simulink model "csu_cmg_camera_geometry_hrn"  (R2014b)
settings: Solver=FixedStepDiscrete  StartTime=0  StopTime=1  FixedStep=1  RelTol=1e-3
values from neighbouring files (symbols this model uses):
  cam_extrinsic_init = zeros(3,4)    [csc_cam_camera_system_init.m]
  cam_image_plane_norm = [0 0 1]    [csc_cam_camera_system_init.m]
  topo_pos_in = [0 0 50+(central_body_radius + ini_alt_wrt_meanrad) ]    [csu_cmg_camera_geometry_test.m]
  topo_q_in = [0 0 sind(5/2) cosd(5/2)]    [csu_cmg_camera_geometry_test.m]
undefined symbols (not defined in the file or in its folder): cam_cam_lander_dcm, cam_intrinsic_matrix_c, cam_position_in_lander, cam_u_matrix, csu_cmg_camera_geometry, csu_cmg_camera_geometry_lib, ini_alt_wrt_1738rad, ini_tgt_landing_mcmf_pos
libraries: util_quat_lib x16, util_frame_rotation_lib x8, rotate_lib x2, util_common_lib x2
settings Model: Creator=escrane  LastModifiedBy=mstewart
settings DataIOCC: SignalLoggingSaveFormat=ModelDataLogs
settings OptimizationCC: ExpressionDepthLimit=2147483647
settings DebuggingCC: UnderspecifiedInitializationDetection=Classic  MergeDetectMultiDrivingBlocksExec=none  FcnCallInpInsideContextMsg=EnableAllAsWarning  StateNameClashWarn=warning

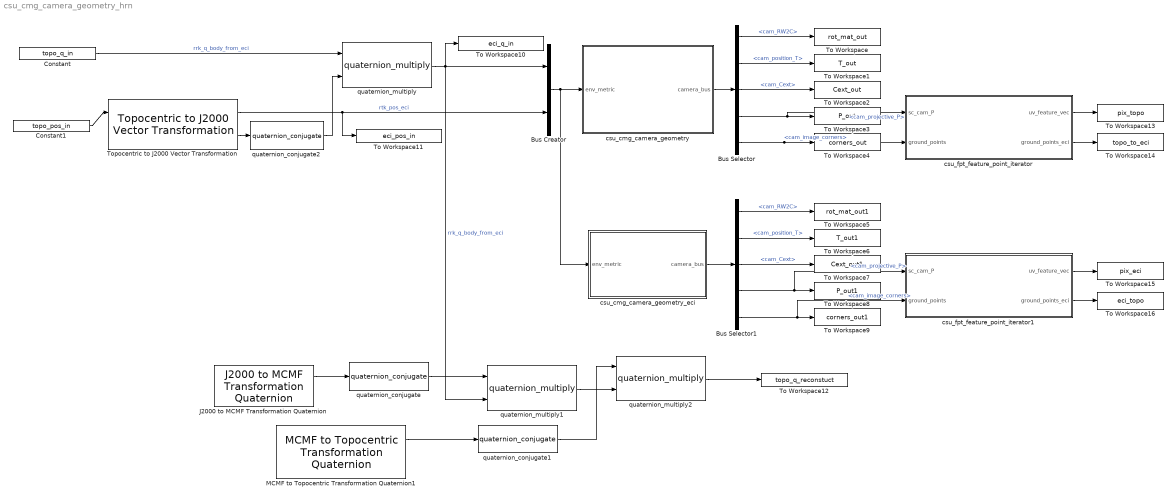
== system csu_cmg_camera_geometry_hrn ==
  Bus Creator : BusCreator  Inputs=2
  Bus Selector : BusSelector  OutputSignals=cam_RW2C,cam_position_T,cam_Cext,cam_projective_P,cam_image_corners
  Bus Selector1 : BusSelector  OutputSignals=cam_RW2C,cam_position_T,cam_Cext,cam_projective_P,cam_image_corners
  Constant : Constant  Value=topo_q_in
  Constant1 : Constant  Value=topo_pos_in
  J2000 to MCMF Transformation Quaternion : util_frame_rotation_lib/J2000 to MCMF  Transformation Quaternion  SystemSampleTime=-1
  MCMF to Topocentric Transformation Quaternion1 : util_frame_rotation_lib/MCMF to Topocentric  Transformation Quaternion  SystemSampleTime=-1
  To Workspace : ToWorkspace  VariableName=rot_mat_out  SaveFormat=Timeseries  SampleTime=-1
  To Workspace1 : ToWorkspace  VariableName=T_out  SaveFormat=Timeseries  SampleTime=-1
  To Workspace10 : ToWorkspace  VariableName=eci_q_in  SaveFormat=Timeseries  SampleTime=-1
  To Workspace11 : ToWorkspace  VariableName=eci_pos_in  SaveFormat=Timeseries  SampleTime=-1
  To Workspace12 : ToWorkspace  VariableName=topo_q_reconstuct  SaveFormat=Timeseries  SampleTime=-1
  To Workspace13 : ToWorkspace  VariableName=pix_topo  SaveFormat=Timeseries  SampleTime=-1
  To Workspace14 : ToWorkspace  VariableName=topo_to_eci  SaveFormat=Timeseries  SampleTime=-1
  To Workspace15 : ToWorkspace  VariableName=pix_eci  SaveFormat=Timeseries  SampleTime=-1
  To Workspace16 : ToWorkspace  VariableName=eci_topo  SaveFormat=Timeseries  SampleTime=-1
  To Workspace2 : ToWorkspace  VariableName=Cext_out  SaveFormat=Timeseries  SampleTime=-1
  To Workspace3 : ToWorkspace  VariableName=P_out  SaveFormat=Timeseries  SampleTime=-1
  To Workspace4 : ToWorkspace  VariableName=corners_out  SaveFormat=Timeseries  SampleTime=-1
  To Workspace5 : ToWorkspace  VariableName=rot_mat_out1  SaveFormat=Timeseries  SampleTime=-1
  To Workspace6 : ToWorkspace  VariableName=T_out1  SaveFormat=Timeseries  SampleTime=-1
  To Workspace7 : ToWorkspace  VariableName=Cext_out1  SaveFormat=Timeseries  SampleTime=-1
  To Workspace8 : ToWorkspace  VariableName=P_out1  SaveFormat=Timeseries  SampleTime=-1
  To Workspace9 : ToWorkspace  VariableName=corners_out1  SaveFormat=Timeseries  SampleTime=-1
  "Topocentric to J2000 Vector Transformation " : util_frame_rotation_lib/Topocentric to J2000 Vector Transformation   SystemSampleTime=-1
  csu_cmg_camera_geometry : Subsystem  AncestorBlock=csu_cmg_camera_geometry_lib/csu_cmg_camera_geometry
  csu_cmg_camera_geometry_eci : Subsystem
  csu_fpt_feature_point_iterator : Subsystem  TreatAsAtomicUnit=on
  csu_fpt_feature_point_iterator1 : Subsystem  TreatAsAtomicUnit=on
  quaternion_conjugate : util_quat_lib/quaternion_conjugate  SystemSampleTime=-1
  quaternion_conjugate1 : util_quat_lib/quaternion_conjugate  SystemSampleTime=-1
  quaternion_conjugate2 : util_quat_lib/quaternion_conjugate  SystemSampleTime=-1
  quaternion_multiply : util_quat_lib/quaternion_multiply  SystemSampleTime=-1
  quaternion_multiply1 : util_quat_lib/quaternion_multiply  SystemSampleTime=-1
  quaternion_multiply2 : util_quat_lib/quaternion_multiply  SystemSampleTime=-1
  wires:
  csu_cmg_camera_geometry/1(camera_bus) -> Bus Selector/1
  Bus Selector/1 -> To Workspace/1  "<cam_RW2C>"
  Bus Selector/2 -> To Workspace1/1  "<cam_position_T>"
  Bus Selector/3 -> To Workspace2/1  "<cam_Cext>"
  Bus Selector/4 -> To Workspace3/1, csu_fpt_feature_point_iterator/1(sc_cam_P)  "<cam_projective_P>"
  Bus Selector/5 -> To Workspace4/1, csu_fpt_feature_point_iterator/2(ground_points)  "<cam_image_corners>"
  "Topocentric to J2000 Vector Transformation "/1 -> Bus Creator/2, To Workspace11/1  "rtk_pos_eci"
  Bus Creator/1 -> csu_cmg_camera_geometry/1(env_metric), csu_cmg_camera_geometry_eci/1(env_metric)
  csu_cmg_camera_geometry_eci/1(camera_bus) -> Bus Selector1/1
  Bus Selector1/1 -> To Workspace5/1  "<cam_RW2C>"
  Bus Selector1/2 -> To Workspace6/1  "<cam_position_T>"
  Bus Selector1/3 -> To Workspace7/1  "<cam_Cext>"
  Bus Selector1/4 -> To Workspace8/1, csu_fpt_feature_point_iterator1/1(sc_cam_P)  "<cam_projective_P>"
  Bus Selector1/5 -> To Workspace9/1, csu_fpt_feature_point_iterator1/2(ground_points)  "<cam_image_corners>"
  Constant1/1 -> "Topocentric to J2000 Vector Transformation "/1
  quaternion_multiply/1 -> Bus Creator/1, To Workspace10/1, quaternion_multiply1/2  "rrk_q_body_from_eci"
  quaternion_conjugate1/1 -> quaternion_multiply2/1
  quaternion_conjugate/1 -> quaternion_multiply1/1
  quaternion_multiply2/1 -> To Workspace12/1
  quaternion_multiply1/1 -> quaternion_multiply2/2
  J2000 to MCMF Transformation Quaternion/1 -> quaternion_conjugate/1
  MCMF to Topocentric Transformation Quaternion1/1 -> quaternion_conjugate1/1
  Constant/1 -> quaternion_multiply/1  "rrk_q_body_from_eci"
  "Topocentric to J2000 Vector Transformation "/2 -> quaternion_conjugate2/1
  quaternion_conjugate2/1 -> quaternion_multiply/2
  csu_fpt_feature_point_iterator/2(ground_points_eci) -> To Workspace14/1
  csu_fpt_feature_point_iterator/1(uv_feature_vec) -> To Workspace13/1
  csu_fpt_feature_point_iterator1/2(ground_points_eci) -> To Workspace16/1
  csu_fpt_feature_point_iterator1/1(uv_feature_vec) -> To Workspace15/1

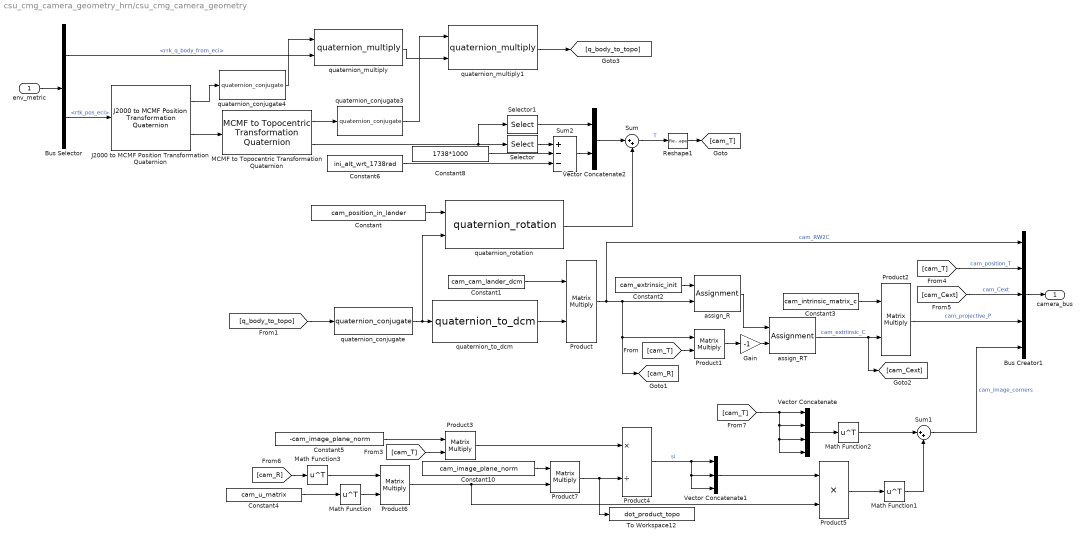
== system csu_cmg_camera_geometry_hrn/csu_cmg_camera_geometry ==
  env_metric : Inport
  Bus Creator1 : BusCreator  Inputs=5
  Bus Selector : BusSelector  OutputSignals=rrk_q_body_from_eci,rtk_pos_eci
  Constant : Constant  Value=cam_position_in_lander
  Constant1 : Constant  Value=cam_cam_lander_dcm
  Constant10 : Constant  Value=cam_image_plane_norm  VectorParams1D=off
  Constant2 : Constant  Value=cam_extrinsic_init
  Constant3 : Constant  Value=cam_intrinsic_matrix_c
  Constant4 : Constant  Value=cam_u_matrix
  Constant5 : Constant  Value=-cam_image_plane_norm  VectorParams1D=off
  Constant6 : Constant  Value=ini_alt_wrt_1738rad
  Constant8 : Constant  Value=1738*1000
  Gain : Gain  Gain=-1
  J2000 to MCMF Position Transformation Quaternion : rotate_lib/J2000 to MCMF Position Transformation Quaternion
  MCMF to Topocentric Transformation Quaternion : util_frame_rotation_lib/MCMF to Topocentric  Transformation Quaternion  SystemSampleTime=-1
  Math Function{,1..3} (4 alike) : Math  Operator=transpose  SaturateOnIntegerOverflow=on
  Product{,1..3,6..7} (6 alike) : Product  Multiplication=Matrix(*)  RndMeth=Zero
  Product4 : Product  Inputs=*/  RndMeth=Zero
  Product5 : Product  Inputs=**  RndMeth=Zero
  Reshape1 : Reshape  OutputDimensionality=Column vector (2-D)
  Selector : Selector  InputPortWidth=3  Indices=[3]
  Selector1 : Selector  InputPortWidth=3  Indices=[1 2]
  Sum : Sum  Inputs=|++
  Sum1 : Sum  Inputs=|++
  Sum2 : Sum  Inputs=+--
  To Workspace12 : ToWorkspace  VariableName=dot_product_topo  SaveFormat=Timeseries  SampleTime=-1
  Vector Concatenate : Concatenate  NumInputs=4  Mode=Multidimensional array  ConcatenateDimension=2
  Vector Concatenate1 : Concatenate  NumInputs=3  Mode=Multidimensional array
  Vector Concatenate2 : Concatenate
  assign_R : Assignment  NumberOfDimensions=2  IndexOptions=Index vector (dialog),Index vector (dialog)  Indices=[1 2 3],[1 2 3]  OutputSizes=1,1
  assign_RT : Assignment  NumberOfDimensions=2  IndexOptions=Index vector (dialog),Index vector (dialog)  Indices=[1 2 3],[4]  OutputSizes=1,1
  quaternion_conjugate : util_quat_lib/quaternion_conjugate  SystemSampleTime=-1
  quaternion_conjugate3 : util_quat_lib/quaternion_conjugate  SystemSampleTime=-1
  quaternion_conjugate4 : util_quat_lib/quaternion_conjugate  SystemSampleTime=-1
  quaternion_multiply : util_quat_lib/quaternion_multiply  SystemSampleTime=-1
  quaternion_multiply1 : util_quat_lib/quaternion_multiply  SystemSampleTime=-1
  quaternion_rotation : util_quat_lib/quaternion_rotation  SystemSampleTime=-1
  quaternion_to_dcm : util_quat_lib/quaternion_to_dcm  SystemSampleTime=-1
  camera_bus : Outport
  wires:
  Bus Creator1/1 -> camera_bus/1
  [cam_Cext] -> Bus Creator1/3  "cam_Cext"
  [cam_T] -> Bus Creator1/2  "cam_position_T"
  Sum1/1 -> Bus Creator1/5  "cam_image_corners"
  Product5/1 -> Math Function1/1
  Product7/1 -> Product4/2, To Workspace12/1
  Product3/1 -> Product4/1
  Constant3/1 -> Product2/1
  Product2/1 -> Bus Creator1/4  "cam_projective_P"
  assign_RT/1 -> [cam_Cext], Product2/2  "cam_extriinsic_C"
  Gain/1 -> assign_RT/2
  Product1/1 -> Gain/1
  assign_R/1 -> assign_RT/1
  [cam_T] -> Product1/2
  Sum/1 -> Reshape1/1  "T"
  Constant2/1 -> assign_R/1
  Product/1 -> Bus Creator1/1, assign_R/2, [cam_R], Product1/1  "cam_RW2C"
  quaternion_rotation/1 -> Sum/2
  Constant/1 -> quaternion_rotation/1
  [q_body_to_topo] -> quaternion_conjugate/1
  Bus Selector/2 -> J2000 to MCMF Position Transformation Quaternion/1  "<rtk_pos_eci>"
  env_metric/1 -> Bus Selector/1
  J2000 to MCMF Position Transformation Quaternion/2 -> MCMF to Topocentric Transformation Quaternion/1
  Product6/1 -> Product5/2, Product7/2
  Constant4/1 -> Math Function/1
  [cam_R] -> Math Function3/1
  Math Function/1 -> Product6/2
  Math Function2/1 -> Sum1/1
  Vector Concatenate/1 -> Math Function2/1
  [cam_T] -> Vector Concatenate/1, Vector Concatenate/2, Vector Concatenate/3, Vector Concatenate/4
  Product4/1 -> Vector Concatenate1/1, Vector Concatenate1/2, Vector Concatenate1/3  "si"
  Vector Concatenate1/1 -> Product5/1
  Reshape1/1 -> [cam_T]
  MCMF to Topocentric Transformation Quaternion/2 -> Selector/1, Selector1/1
  Constant6/1 -> Sum2/3
  Constant8/1 -> Sum2/2
  Selector1/1 -> Vector Concatenate2/1
  Selector/1 -> Sum2/1
  Sum2/1 -> Vector Concatenate2/2
  Vector Concatenate2/1 -> Sum/1
  quaternion_multiply1/1 -> [q_body_to_topo]
  Math Function3/1 -> Product6/1
  Constant5/1 -> Product3/1
  [cam_T] -> Product3/2
  Constant10/1 -> Product7/1
  Math Function1/1 -> Sum1/2
  quaternion_conjugate/1 -> quaternion_rotation/2, quaternion_to_dcm/1
  MCMF to Topocentric Transformation Quaternion/1 -> quaternion_conjugate3/1
  quaternion_conjugate3/1 -> quaternion_multiply1/1
  quaternion_multiply/1 -> quaternion_multiply1/2
  J2000 to MCMF Position Transformation Quaternion/1 -> quaternion_conjugate4/1
  Bus Selector/1 -> quaternion_multiply/2  "<rrk_q_body_from_eci>"
  quaternion_conjugate4/1 -> quaternion_multiply/1
  Constant1/1 -> Product/1
  quaternion_to_dcm/1 -> Product/2

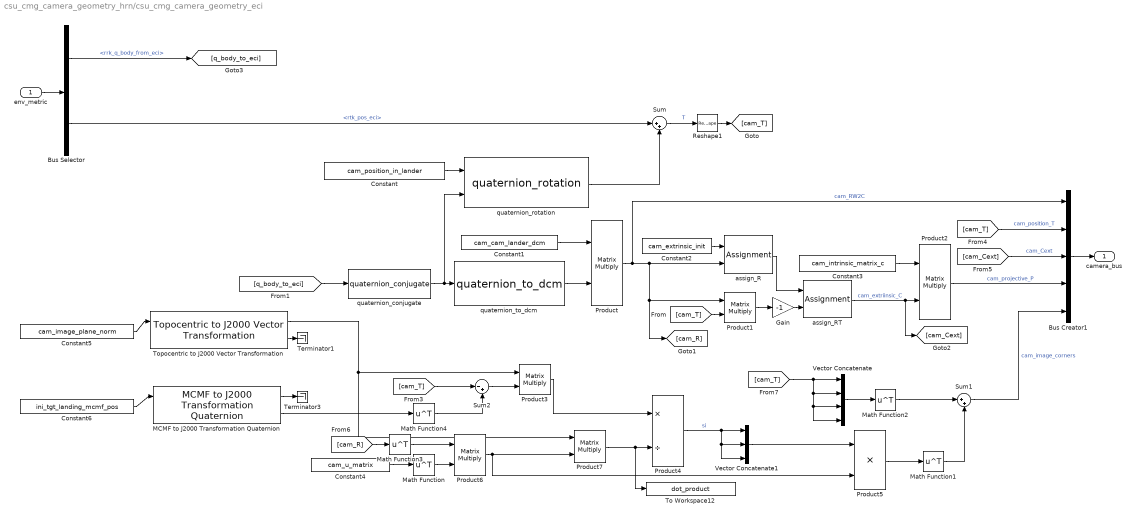
== system csu_cmg_camera_geometry_hrn/csu_cmg_camera_geometry_eci ==
  env_metric : Inport
  Bus Creator1 : BusCreator  Inputs=5
  Bus Selector : BusSelector  OutputSignals=rrk_q_body_from_eci,rtk_pos_eci
  Constant : Constant  Value=cam_position_in_lander
  Constant1 : Constant  Value=cam_cam_lander_dcm
  Constant2 : Constant  Value=cam_extrinsic_init
  Constant3 : Constant  Value=cam_intrinsic_matrix_c
  Constant4 : Constant  Value=cam_u_matrix
  Constant5 : Constant  Value=cam_image_plane_norm  VectorParams1D=off
  Constant6 : Constant  Value=ini_tgt_landing_mcmf_pos  VectorParams1D=off
  Gain : Gain  Gain=-1
  MCMF to J2000 Transformation Quaternion : util_frame_rotation_lib/MCMF to J2000  Transformation Quaternion
  Math Function{,1..4} (5 alike) : Math  Operator=transpose  SaturateOnIntegerOverflow=on
  Product{,1..3,6..7} (6 alike) : Product  Multiplication=Matrix(*)  RndMeth=Zero
  Product4 : Product  Inputs=*/  RndMeth=Zero
  Product5 : Product  Inputs=**  RndMeth=Zero
  Reshape1 : Reshape  OutputDimensionality=Column vector (2-D)
  Sum : Sum  Inputs=|++
  Sum1 : Sum  Inputs=|++
  Sum2 : Sum  Inputs=|-+
  Terminator1 : Terminator
  Terminator3 : Terminator
  To Workspace12 : ToWorkspace  VariableName=dot_product  SaveFormat=Timeseries  SampleTime=-1
  "Topocentric to J2000 Vector Transformation " : util_frame_rotation_lib/Topocentric to J2000 Vector Transformation   SystemSampleTime=-1
  Vector Concatenate : Concatenate  NumInputs=4  Mode=Multidimensional array  ConcatenateDimension=2
  Vector Concatenate1 : Concatenate  NumInputs=3  Mode=Multidimensional array
  assign_R : Assignment  NumberOfDimensions=2  IndexOptions=Index vector (dialog),Index vector (dialog)  Indices=[1 2 3],[1 2 3]  OutputSizes=1,1
  assign_RT : Assignment  NumberOfDimensions=2  IndexOptions=Index vector (dialog),Index vector (dialog)  Indices=[1 2 3],[4]  OutputSizes=1,1
  quaternion_conjugate : util_quat_lib/quaternion_conjugate  SystemSampleTime=-1
  quaternion_rotation : util_quat_lib/quaternion_rotation  SystemSampleTime=-1
  quaternion_to_dcm : util_quat_lib/quaternion_to_dcm  SystemSampleTime=-1
  camera_bus : Outport
  wires:
  Bus Creator1/1 -> camera_bus/1
  [cam_Cext] -> Bus Creator1/3  "cam_Cext"
  [cam_T] -> Bus Creator1/2  "cam_position_T"
  Sum1/1 -> Bus Creator1/5  "cam_image_corners"
  Product5/1 -> Math Function1/1
  Product7/1 -> Product4/2, To Workspace12/1
  Product3/1 -> Product4/1
  Constant3/1 -> Product2/1
  Product2/1 -> Bus Creator1/4  "cam_projective_P"
  assign_RT/1 -> [cam_Cext], Product2/2  "cam_extriinsic_C"
  Gain/1 -> assign_RT/2
  Product1/1 -> Gain/1
  assign_R/1 -> assign_RT/1
  [cam_T] -> Product1/2
  Sum/1 -> Reshape1/1  "T"
  Constant2/1 -> assign_R/1
  Product/1 -> Bus Creator1/1, assign_R/2, [cam_R], Product1/1  "cam_RW2C"
  quaternion_rotation/1 -> Sum/2
  Constant/1 -> quaternion_rotation/1
  [q_body_to_eci] -> quaternion_conjugate/1
  Bus Selector/2 -> Sum/1  "<rtk_pos_eci>"
  env_metric/1 -> Bus Selector/1
  Product6/1 -> Product7/2, Product5/2
  Constant4/1 -> Math Function/1
  [cam_R] -> Math Function3/1
  Math Function/1 -> Product6/2
  Math Function2/1 -> Sum1/1
  Vector Concatenate/1 -> Math Function2/1
  [cam_T] -> Vector Concatenate/1, Vector Concatenate/2, Vector Concatenate/3, Vector Concatenate/4
  Product4/1 -> Vector Concatenate1/1, Vector Concatenate1/2, Vector Concatenate1/3  "si"
  Vector Concatenate1/1 -> Product5/1
  Reshape1/1 -> [cam_T]
  Math Function3/1 -> Product6/1
  Math Function1/1 -> Sum1/2
  Bus Selector/1 -> [q_body_to_eci]  "<rrk_q_body_from_eci>"
  [cam_T] -> Sum2/1
  Sum2/1 -> Product3/2
  Constant6/1 -> MCMF to J2000 Transformation Quaternion/1
  MCMF to J2000 Transformation Quaternion/2 -> Math Function4/1
  MCMF to J2000 Transformation Quaternion/1 -> Terminator3/1
  Constant5/1 -> "Topocentric to J2000 Vector Transformation "/1
  "Topocentric to J2000 Vector Transformation "/1 -> Product3/1, Product7/1
  Math Function4/1 -> Sum2/2
  quaternion_conjugate/1 -> quaternion_rotation/2, quaternion_to_dcm/1
  "Topocentric to J2000 Vector Transformation "/2 -> Terminator1/1
  Constant1/1 -> Product/1
  quaternion_to_dcm/1 -> Product/2

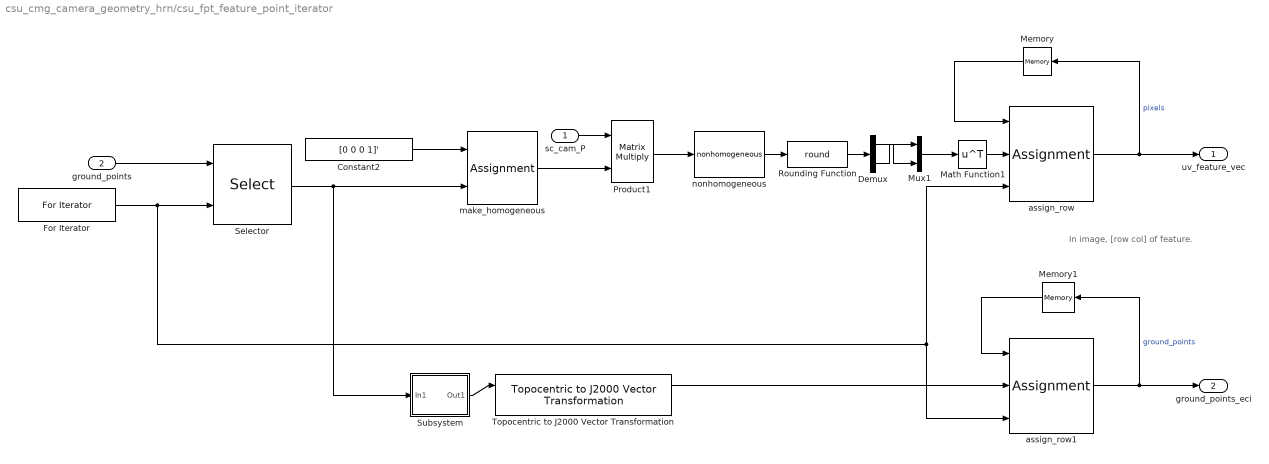
== system csu_cmg_camera_geometry_hrn/csu_fpt_feature_point_iterator ==
  note: In image, [row col] of feature.
  sc_cam_P : Inport
  ground_points : Inport  Port=2
  Constant2 : Constant  Value=[0 0 0 1]'  VectorParams1D=off
  Demux : Demux  Outputs=2
  For Iterator : ForIterator  IterationLimit=4
  Math Function1 : Math  Operator=transpose  SaturateOnIntegerOverflow=on
  Memory : Memory  X0=zeros(4,2)  InheritSampleTime=on
  Memory1 : Memory  X0=zeros(4,3)  InheritSampleTime=on
  Mux1 : Mux  Inputs=2
  Product1 : Product  Multiplication=Matrix(*)  RndMeth=Zero
  Rounding Function : Rounding  Operator=round
  Selector : Selector  NumberOfDimensions=2  InputPortWidth=[10 2]  IndexOptions=Index vector (port),Select all  Indices=[1 3],1  OutputSizes=1,1
  Subsystem : Subsystem
  "Topocentric to J2000 Vector Transformation " : util_frame_rotation_lib/Topocentric to J2000 Vector Transformation   SystemSampleTime=-1
  assign_row : Assignment  NumberOfDimensions=2  IndexOptions=Index vector (port),Assign all  Indices=1,1  OutputSizes=1,1
  assign_row1 : Assignment  NumberOfDimensions=2  IndexOptions=Index vector (port),Assign all  Indices=1,1  OutputSizes=1,1
  make_homogeneous : Assignment  Indices=[1 2 3]
  nonhomogeneous : util_common_lib/nonhomogeneous  SystemSampleTime=-1
  uv_feature_vec : Outport
  ground_points_eci : Outport  Port=2
  wires:
  Memory/1 -> assign_row/1
  assign_row/1 -> Memory/1, uv_feature_vec/1  "pixels"
  For Iterator/1 -> Selector/2, assign_row/3, assign_row1/3
  ground_points/1 -> Selector/1
  nonhomogeneous/1 -> Rounding Function/1
  Product1/1 -> nonhomogeneous/1
  make_homogeneous/1 -> Product1/2
  sc_cam_P/1 -> Product1/1
  Constant2/1 -> make_homogeneous/1
  Math Function1/1 -> assign_row/2
  Rounding Function/1 -> Demux/1
  Mux1/1 -> Math Function1/1
  Demux/2 -> Mux1/1
  Demux/1 -> Mux1/2
  assign_row1/1 -> ground_points_eci/1, Memory1/1  "ground_points"
  Memory1/1 -> assign_row1/1
  Selector/1 -> make_homogeneous/2, Subsystem/1(In1)
  Subsystem/1(Out1) -> "Topocentric to J2000 Vector Transformation "/1
  "Topocentric to J2000 Vector Transformation "/1 -> assign_row1/2

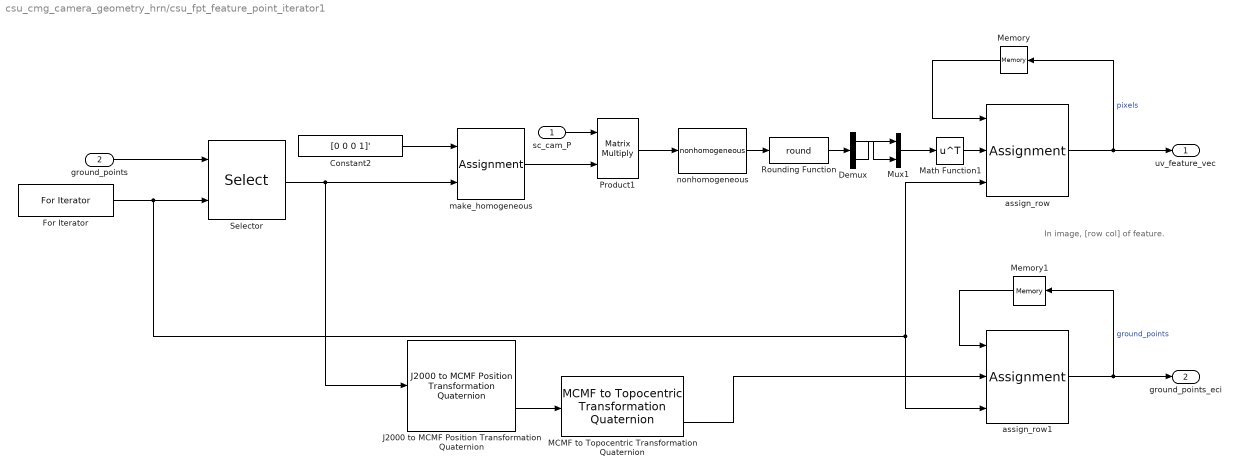
== system csu_cmg_camera_geometry_hrn/csu_fpt_feature_point_iterator1 ==
  note: In image, [row col] of feature.
  sc_cam_P : Inport
  ground_points : Inport  Port=2
  Constant2 : Constant  Value=[0 0 0 1]'  VectorParams1D=off
  Demux : Demux  Outputs=2
  For Iterator : ForIterator  IterationLimit=4
  J2000 to MCMF Position Transformation Quaternion : rotate_lib/J2000 to MCMF Position Transformation Quaternion
  MCMF to Topocentric Transformation Quaternion : util_frame_rotation_lib/MCMF to Topocentric  Transformation Quaternion  SystemSampleTime=-1
  Math Function1 : Math  Operator=transpose  SaturateOnIntegerOverflow=on
  Memory : Memory  X0=zeros(4,2)  InheritSampleTime=on
  Memory1 : Memory  X0=zeros(4,3)  InheritSampleTime=on
  Mux1 : Mux  Inputs=2
  Product1 : Product  Multiplication=Matrix(*)  RndMeth=Zero
  Rounding Function : Rounding  Operator=round
  Selector : Selector  NumberOfDimensions=2  InputPortWidth=[10 2]  IndexOptions=Index vector (port),Select all  Indices=[1 3],1  OutputSizes=1,1
  assign_row : Assignment  NumberOfDimensions=2  IndexOptions=Index vector (port),Assign all  Indices=1,1  OutputSizes=1,1
  assign_row1 : Assignment  NumberOfDimensions=2  IndexOptions=Index vector (port),Assign all  Indices=1,1  OutputSizes=1,1
  make_homogeneous : Assignment  Indices=[1 2 3]
  nonhomogeneous : util_common_lib/nonhomogeneous  SystemSampleTime=-1
  uv_feature_vec : Outport
  ground_points_eci : Outport  Port=2
  wires:
  Memory/1 -> assign_row/1
  assign_row/1 -> Memory/1, uv_feature_vec/1  "pixels"
  For Iterator/1 -> Selector/2, assign_row/3, assign_row1/3
  ground_points/1 -> Selector/1
  nonhomogeneous/1 -> Rounding Function/1
  Product1/1 -> nonhomogeneous/1
  make_homogeneous/1 -> Product1/2
  sc_cam_P/1 -> Product1/1
  Constant2/1 -> make_homogeneous/1
  Math Function1/1 -> assign_row/2
  Rounding Function/1 -> Demux/1
  Mux1/1 -> Math Function1/1
  Demux/2 -> Mux1/1
  Demux/1 -> Mux1/2
  assign_row1/1 -> ground_points_eci/1, Memory1/1  "ground_points"
  Memory1/1 -> assign_row1/1
  Selector/1 -> make_homogeneous/2, J2000 to MCMF Position Transformation Quaternion/1
  J2000 to MCMF Position Transformation Quaternion/2 -> MCMF to Topocentric Transformation Quaternion/1
  MCMF to Topocentric Transformation Quaternion/2 -> assign_row1/2

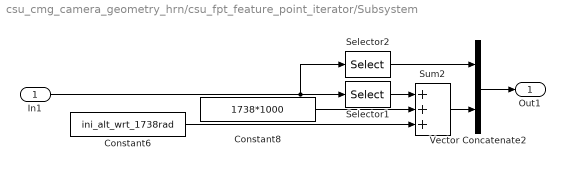
== system csu_cmg_camera_geometry_hrn/csu_fpt_feature_point_iterator/Subsystem ==
  In1 : Inport
  Constant6 : Constant  Value=ini_alt_wrt_1738rad
  Constant8 : Constant  Value=1738*1000
  Selector1 : Selector  InputPortWidth=3  Indices=[3]
  Selector2 : Selector  InputPortWidth=3  Indices=[1 2]
  Sum2 : Sum  Inputs=+++
  Vector Concatenate2 : Concatenate
  Out1 : Outport
  wires:
  In1/1 -> Selector1/1, Selector2/1
  Constant6/1 -> Sum2/3
  Constant8/1 -> Sum2/2
  Selector2/1 -> Vector Concatenate2/1
  Selector1/1 -> Sum2/1
  Sum2/1 -> Vector Concatenate2/2
  Vector Concatenate2/1 -> Out1/1
